simulink model "test_bu01_2018b_tuning"  (R2018b)
settings: Solver=FixedStepAuto  StartTime=0.0  StopTime=10  FixedStep=0.001  RelTol=1e-3
model workspace (MAT data in the model file):
  B1 = 0.0229925610147
  B2 = -0.371283802987
  B3 = -0.920624315565
  B4 = -0.0418343375444
  B5 = -0.493210333206
  B6 = 0
  B7 = -0.0892006103314
  B8 = -0.433620647544
  Ixx = 0.8
  Iyy = 2.075
  Izz = 1.25
  K = 0.92
  K1 = 0.96
  M1 = [1 1 -1 0.151123095698]
  M2 = [1 0 1 0.728919165533]
  M3 = [-1 0 -1 0]
  M4 = [-1 1 1 0.279370204784]
  M5 = [0 -1 0 0.953177368176]
  M6 = [0 -1 0 -1]
  M7 = [0 -1 0 0.164756597211]
  M8 = [0 -1 0 0.72330475505]
  Mass = 11.5
  b = 0
libraries: simulink x4, vrlib x4, shared6dof x1
(part 2 of 3)

== system test_bu01_2018b_tuning/Plant/bu01_model/动力系统模型/Motor4_TM_N/TMU5KV400 /DCMotor1 ==
  In1 : Inport
  Add : Sum  Inputs=+--
  Add1 : Sum  Inputs=+-
  Add2 : Sum
  Add3 : Sum  Inputs=+-
  Bus Selector : BusSelector  OutputSignals=Um,Tq,Izz
  Bus Creator : BusCreator  Inputs=2
  Constant : Constant  Value=Imzz
  Constant1 : Constant  Value=I0
  Divide : Product  Inputs=*/
  Gain : Gain  Gain=1/L
  Gain1 : Gain  Gain=Km
  Gain3 : Gain  Gain=Kemf
  Gain4 : Gain  Gain=Ra
  Gain5 : Gain  Gain=1/(2*pi)
  Gain6 : Gain  Gain=60
  Integrator : Integrator  InitialCondition=0.0001
  Integrator1 : Integrator  InitialCondition=0.0001
  Multiply : Product
  Multiply1 : Product
  Terminator : Terminator
  Terminator1 : Terminator
  Out1 : Outport
  wires:
  In1/1 -> Bus Selector/1
  Bus Selector/1 -> Multiply/1, Add/1  "<Um>"
  Add/1 -> Gain/1
  Gain/1 -> Integrator/1
  Integrator/1 -> Add3/1, Multiply/2, Bus Creator/1, Gain4/1  "Im"
  Gain1/1 -> Multiply1/1, Add1/1  "Te"
  Integrator1/1 -> Multiply1/2, Gain3/1, Gain5/1  "w"
  Add1/1 -> Divide/1
  Divide/1 -> Integrator1/1
  Gain3/1 -> Add/2  "Ea"
  Gain4/1 -> Add/3
  Bus Selector/2 -> [Tq]  "<Tq>"
  Bus Selector/3 -> Add2/1  "<Izz>"
  Constant/1 -> Add2/2
  Add2/1 -> [J]
  [J] -> Divide/2
  Multiply/1 -> Terminator/1  "Pwin"
  Multiply1/1 -> Terminator1/1  "Pwout"
  Gain5/1 -> Gain6/1  "RPS"
  Gain6/1 -> Bus Creator/2  "RPM"
  Bus Creator/1 -> Out1/1
  [Tq] -> Add1/2
  Add3/1 -> Gain1/1  "Iav"
  Constant1/1 -> Add3/2

== system test_bu01_2018b_tuning/Plant/bu01_model/动力系统模型/Motor5_PF_N/PF70mmDuctFanN/涵道风扇模型  ==
  In1 : Inport
  Bus Creator : BusCreator  Inputs=7
  Bus Selector : BusSelector  OutputSignals=Vb,Wb,Ax,Ns,Pro
  If : If  IfExpression=u1 > 1
  Merge : Merge
  Sum : Sum  Inputs=|+-
  Sum1 : Sum  Inputs=|+-
  Terminator : Terminator
  Va : Sqrt  SaturateOnIntegerOverflow=on
  Va^2 : DotProduct  InputSameDT=on  OutDataTypeStr=Inherit: Inherit via internal rule
  Vha : Sqrt  SaturateOnIntegerOverflow=on
  Vva : DotProduct  InputSameDT=on  OutDataTypeStr=Inherit: Inherit via internal rule
  Vva1 : UnaryMinus
  Vva^2 : Math  Operator=square  SaturateOnIntegerOverflow=on
  "[Uba,Vba,Wba]" : UnaryMinus
  求解涵道风扇气动载荷 : Subsystem  TreatAsAtomicUnit=on
  转速太低无载荷输出 : Subsystem  TreatAsAtomicUnit=on
  Out1 : Outport
  wires:
  Bus Selector/1 -> Sum/1  "<Vb>"
  In1/1 -> Bus Selector/1
  Bus Selector/2 -> Sum/2  "<Wb>"
  Sum/1 -> "[Uba,Vba,Wba]"/1
  "[Uba,Vba,Wba]"/1 -> Bus Creator/1, Vva/1, Va^2/2, Va^2/1  "Vba"
  Bus Selector/3 -> Bus Creator/4, Vva/2  "<Ax>"
  Va^2/1 -> Sum1/1, Va/1
  Vva/1 -> Bus Creator/7, Vva^2/1, Vva1/1  "Vva"
  Vva^2/1 -> Sum1/2
  Sum1/1 -> Vha/1
  Vha/1 -> Bus Creator/2  "Vha"
  Vva1/1 -> Bus Creator/3  "Vva1"
  Bus Selector/4 -> Bus Creator/5, If/1  "<Ns>"
  If/1 -> 求解涵道风扇气动载荷/Action
  If/2 -> 转速太低无载荷输出/Action
  Bus Selector/5 -> Bus Creator/6  "<Pro>"
  Bus Creator/1 -> 求解涵道风扇气动载荷/1(In1)
  求解涵道风扇气动载荷/1(Out1) -> Merge/1  "Fb&Mb"
  转速太低无载荷输出/1(Out1) -> Merge/2  "Fb&Mb"
  Va/1 -> Terminator/1  "Va"
  Merge/1 -> Out1/1  "Fb&Mb"

== system test_bu01_2018b_tuning/Plant/bu01_model/动力系统模型/Motor5_PF_N/PFKV2300/DCMotor ==
  In1 : Inport
  Add : Sum  Inputs=+--
  Add1 : Sum  Inputs=+-
  Add2 : Sum
  Add3 : Sum  Inputs=+-
  Bus Selector : BusSelector  OutputSignals=Um,Tq,Izz
  Bus Creator : BusCreator  Inputs=2
  Constant : Constant  Value=Imzz
  Constant1 : Constant  Value=I0
  Divide : Product  Inputs=*/
  Gain : Gain  Gain=1/L
  Gain1 : Gain  Gain=Km
  Gain3 : Gain  Gain=Kemf
  Gain4 : Gain  Gain=Ra
  Gain5 : Gain  Gain=1/(2*pi)
  Gain6 : Gain  Gain=60
  Integrator : Integrator
  Integrator1 : Integrator
  Multiply : Product
  Multiply1 : Product
  Terminator : Terminator
  Terminator1 : Terminator
  Out1 : Outport
  wires:
  In1/1 -> Bus Selector/1
  Bus Selector/1 -> Multiply/1, Add/1  "<Um>"
  Add/1 -> Gain/1
  Gain/1 -> Integrator/1
  Integrator/1 -> Add3/1, Multiply/2, Bus Creator/1, Gain4/1  "Im"
  Gain1/1 -> Multiply1/1, Add1/1  "Te"
  Integrator1/1 -> Multiply1/2, Gain3/1, Gain5/1  "w"
  Add1/1 -> Divide/1
  Divide/1 -> Integrator1/1
  Gain3/1 -> Add/2  "Ea"
  Gain4/1 -> Add/3
  Bus Selector/2 -> [Tq]  "<Tq>"
  Bus Selector/3 -> Add2/1  "<Izz>"
  Constant/1 -> Add2/2
  Add2/1 -> [J]
  [J] -> Divide/2
  Multiply/1 -> Terminator/1  "Pwin"
  Multiply1/1 -> Terminator1/1  "Pwout"
  Gain5/1 -> Gain6/1  "RPS"
  Gain6/1 -> Bus Creator/2  "RPM"
  Bus Creator/1 -> Out1/1
  [Tq] -> Add1/2
  Add3/1 -> Gain1/1  "Iav"
  Constant1/1 -> Add3/2

== system test_bu01_2018b_tuning/Plant/bu01_model/动力系统模型/Motor6_PF_N/PF70mmDuctFanN/涵道风扇模型  ==
  In1 : Inport
  Bus Creator : BusCreator  Inputs=7
  Bus Selector : BusSelector  OutputSignals=Vb,Wb,Ax,Ns,Pro
  If : If  IfExpression=u1 > 1
  Merge : Merge
  Sum : Sum  Inputs=|+-
  Sum1 : Sum  Inputs=|+-
  Terminator : Terminator
  Va : Sqrt  SaturateOnIntegerOverflow=on
  Va^2 : DotProduct  InputSameDT=on  OutDataTypeStr=Inherit: Inherit via internal rule
  Vha : Sqrt  SaturateOnIntegerOverflow=on
  Vva : DotProduct  InputSameDT=on  OutDataTypeStr=Inherit: Inherit via internal rule
  Vva1 : UnaryMinus
  Vva^2 : Math  Operator=square  SaturateOnIntegerOverflow=on
  "[Uba,Vba,Wba]" : UnaryMinus
  求解涵道风扇气动载荷 : Subsystem  TreatAsAtomicUnit=on
  转速太低无载荷输出 : Subsystem  TreatAsAtomicUnit=on
  Out1 : Outport
  wires:
  Bus Selector/1 -> Sum/1  "<Vb>"
  In1/1 -> Bus Selector/1
  Bus Selector/2 -> Sum/2  "<Wb>"
  Sum/1 -> "[Uba,Vba,Wba]"/1
  "[Uba,Vba,Wba]"/1 -> Bus Creator/1, Vva/1, Va^2/2, Va^2/1  "Vba"
  Bus Selector/3 -> Bus Creator/4, Vva/2  "<Ax>"
  Va^2/1 -> Sum1/1, Va/1
  Vva/1 -> Bus Creator/7, Vva^2/1, Vva1/1  "Vva"
  Vva^2/1 -> Sum1/2
  Sum1/1 -> Vha/1
  Vha/1 -> Bus Creator/2  "Vha"
  Vva1/1 -> Bus Creator/3  "Vva1"
  Bus Selector/4 -> Bus Creator/5, If/1  "<Ns>"
  If/1 -> 求解涵道风扇气动载荷/Action
  If/2 -> 转速太低无载荷输出/Action
  Bus Selector/5 -> Bus Creator/6  "<Pro>"
  Bus Creator/1 -> 求解涵道风扇气动载荷/1(In1)
  求解涵道风扇气动载荷/1(Out1) -> Merge/1  "Fb&Mb"
  转速太低无载荷输出/1(Out1) -> Merge/2  "Fb&Mb"
  Va/1 -> Terminator/1  "Va"
  Merge/1 -> Out1/1  "Fb&Mb"

== system test_bu01_2018b_tuning/Plant/bu01_model/动力系统模型/Motor6_PF_N/PFKV2300/DCMotor ==
  In1 : Inport
  Add : Sum  Inputs=+--
  Add1 : Sum  Inputs=+-
  Add2 : Sum
  Add3 : Sum  Inputs=+-
  Bus Selector : BusSelector  OutputSignals=Um,Tq,Izz
  Bus Creator : BusCreator  Inputs=2
  Constant : Constant  Value=Imzz
  Constant1 : Constant  Value=I0
  Divide : Product  Inputs=*/
  Gain : Gain  Gain=1/L
  Gain1 : Gain  Gain=Km
  Gain3 : Gain  Gain=Kemf
  Gain4 : Gain  Gain=Ra
  Gain5 : Gain  Gain=1/(2*pi)
  Gain6 : Gain  Gain=60
  Integrator : Integrator
  Integrator1 : Integrator
  Multiply : Product
  Multiply1 : Product
  Terminator : Terminator
  Terminator1 : Terminator
  Out1 : Outport
  wires:
  In1/1 -> Bus Selector/1
  Bus Selector/1 -> Multiply/1, Add/1  "<Um>"
  Add/1 -> Gain/1
  Gain/1 -> Integrator/1
  Integrator/1 -> Add3/1, Multiply/2, Bus Creator/1, Gain4/1  "Im"
  Gain1/1 -> Multiply1/1, Add1/1  "Te"
  Integrator1/1 -> Multiply1/2, Gain3/1, Gain5/1  "w"
  Add1/1 -> Divide/1
  Divide/1 -> Integrator1/1
  Gain3/1 -> Add/2  "Ea"
  Gain4/1 -> Add/3
  Bus Selector/2 -> [Tq]  "<Tq>"
  Bus Selector/3 -> Add2/1  "<Izz>"
  Constant/1 -> Add2/2
  Add2/1 -> [J]
  [J] -> Divide/2
  Multiply/1 -> Terminator/1  "Pwin"
  Multiply1/1 -> Terminator1/1  "Pwout"
  Gain5/1 -> Gain6/1  "RPS"
  Gain6/1 -> Bus Creator/2  "RPM"
  Bus Creator/1 -> Out1/1
  [Tq] -> Add1/2
  Add3/1 -> Gain1/1  "Iav"
  Constant1/1 -> Add3/2

== system test_bu01_2018b_tuning/Plant/bu01_model/动力系统模型/Motor7_PF_N/PF70mmDuctFanN/涵道风扇模型  ==
  In1 : Inport
  Bus Creator : BusCreator  Inputs=7
  Bus Selector : BusSelector  OutputSignals=Vb,Wb,Ax,Ns,Pro
  If : If  IfExpression=u1 > 1
  Merge : Merge
  Sum : Sum  Inputs=|+-
  Sum1 : Sum  Inputs=|+-
  Terminator : Terminator
  Va : Sqrt  SaturateOnIntegerOverflow=on
  Va^2 : DotProduct  InputSameDT=on  OutDataTypeStr=Inherit: Inherit via internal rule
  Vha : Sqrt  SaturateOnIntegerOverflow=on
  Vva : DotProduct  InputSameDT=on  OutDataTypeStr=Inherit: Inherit via internal rule
  Vva1 : UnaryMinus
  Vva^2 : Math  Operator=square  SaturateOnIntegerOverflow=on
  "[Uba,Vba,Wba]" : UnaryMinus
  求解涵道风扇气动载荷 : Subsystem  TreatAsAtomicUnit=on
  转速太低无载荷输出 : Subsystem  TreatAsAtomicUnit=on
  Out1 : Outport
  wires:
  Bus Selector/1 -> Sum/1  "<Vb>"
  In1/1 -> Bus Selector/1
  Bus Selector/2 -> Sum/2  "<Wb>"
  Sum/1 -> "[Uba,Vba,Wba]"/1
  "[Uba,Vba,Wba]"/1 -> Bus Creator/1, Vva/1, Va^2/2, Va^2/1  "Vba"
  Bus Selector/3 -> Bus Creator/4, Vva/2  "<Ax>"
  Va^2/1 -> Sum1/1, Va/1
  Vva/1 -> Bus Creator/7, Vva^2/1, Vva1/1  "Vva"
  Vva^2/1 -> Sum1/2
  Sum1/1 -> Vha/1
  Vha/1 -> Bus Creator/2  "Vha"
  Vva1/1 -> Bus Creator/3  "Vva1"
  Bus Selector/4 -> Bus Creator/5, If/1  "<Ns>"
  If/1 -> 求解涵道风扇气动载荷/Action
  If/2 -> 转速太低无载荷输出/Action
  Bus Selector/5 -> Bus Creator/6  "<Pro>"
  Bus Creator/1 -> 求解涵道风扇气动载荷/1(In1)
  求解涵道风扇气动载荷/1(Out1) -> Merge/1  "Fb&Mb"
  转速太低无载荷输出/1(Out1) -> Merge/2  "Fb&Mb"
  Va/1 -> Terminator/1  "Va"
  Merge/1 -> Out1/1  "Fb&Mb"

== system test_bu01_2018b_tuning/Plant/bu01_model/动力系统模型/Motor7_PF_N/PFKV2300/DCMotor ==
  In1 : Inport
  Add : Sum  Inputs=+--
  Add1 : Sum  Inputs=+-
  Add2 : Sum
  Add3 : Sum  Inputs=+-
  Bus Selector : BusSelector  OutputSignals=Um,Tq,Izz
  Bus Creator : BusCreator  Inputs=2
  Constant : Constant  Value=Imzz
  Constant1 : Constant  Value=I0
  Divide : Product  Inputs=*/
  Gain : Gain  Gain=1/L
  Gain1 : Gain  Gain=Km
  Gain3 : Gain  Gain=Kemf
  Gain4 : Gain  Gain=Ra
  Gain5 : Gain  Gain=1/(2*pi)
  Gain6 : Gain  Gain=60
  Integrator : Integrator
  Integrator1 : Integrator
  Multiply : Product
  Multiply1 : Product
  Terminator : Terminator
  Terminator1 : Terminator
  Out1 : Outport
  wires:
  In1/1 -> Bus Selector/1
  Bus Selector/1 -> Multiply/1, Add/1  "<Um>"
  Add/1 -> Gain/1
  Gain/1 -> Integrator/1
  Integrator/1 -> Add3/1, Multiply/2, Bus Creator/1, Gain4/1  "Im"
  Gain1/1 -> Multiply1/1, Add1/1  "Te"
  Integrator1/1 -> Multiply1/2, Gain3/1, Gain5/1  "w"
  Add1/1 -> Divide/1
  Divide/1 -> Integrator1/1
  Gain3/1 -> Add/2  "Ea"
  Gain4/1 -> Add/3
  Bus Selector/2 -> [Tq]  "<Tq>"
  Bus Selector/3 -> Add2/1  "<Izz>"
  Constant/1 -> Add2/2
  Add2/1 -> [J]
  [J] -> Divide/2
  Multiply/1 -> Terminator/1  "Pwin"
  Multiply1/1 -> Terminator1/1  "Pwout"
  Gain5/1 -> Gain6/1  "RPS"
  Gain6/1 -> Bus Creator/2  "RPM"
  Bus Creator/1 -> Out1/1
  [Tq] -> Add1/2
  Add3/1 -> Gain1/1  "Iav"
  Constant1/1 -> Add3/2

== system test_bu01_2018b_tuning/Plant/bu01_model/动力系统模型/Motor8_PF_N/PF70mmDuctFanN/涵道风扇模型  ==
  In1 : Inport
  Bus Creator : BusCreator  Inputs=7
  Bus Selector : BusSelector  OutputSignals=Vb,Wb,Ax,Ns,Pro
  If : If  IfExpression=u1 > 1
  Merge : Merge
  Sum : Sum  Inputs=|+-
  Sum1 : Sum  Inputs=|+-
  Terminator : Terminator
  Va : Sqrt  SaturateOnIntegerOverflow=on
  Va^2 : DotProduct  InputSameDT=on  OutDataTypeStr=Inherit: Inherit via internal rule
  Vha : Sqrt  SaturateOnIntegerOverflow=on
  Vva : DotProduct  InputSameDT=on  OutDataTypeStr=Inherit: Inherit via internal rule
  Vva1 : UnaryMinus
  Vva^2 : Math  Operator=square  SaturateOnIntegerOverflow=on
  "[Uba,Vba,Wba]" : UnaryMinus
  求解涵道风扇气动载荷 : Subsystem  TreatAsAtomicUnit=on
  转速太低无载荷输出 : Subsystem  TreatAsAtomicUnit=on
  Out1 : Outport
  wires:
  Merge/1 -> Out1/1  "Fb&Mb"
  Va/1 -> Terminator/1  "Va"
  转速太低无载荷输出/1(Out1) -> Merge/2  "Fb&Mb"
  求解涵道风扇气动载荷/1(Out1) -> Merge/1  "Fb&Mb"
  Bus Creator/1 -> 求解涵道风扇气动载荷/1(In1)
  Bus Selector/5 -> Bus Creator/6  "<Pro>"
  If/2 -> 转速太低无载荷输出/Action
  If/1 -> 求解涵道风扇气动载荷/Action
  Bus Selector/4 -> If/1, Bus Creator/5  "<Ns>"
  Vva1/1 -> Bus Creator/3  "Vva1"
  Vha/1 -> Bus Creator/2  "Vha"
  Sum1/1 -> Vha/1
  Vva^2/1 -> Sum1/2
  Vva/1 -> Vva1/1, Vva^2/1, Bus Creator/7  "Vva"
  Va^2/1 -> Va/1, Sum1/1
  Bus Selector/3 -> Vva/2, Bus Creator/4  "<Ax>"
  "[Uba,Vba,Wba]"/1 -> Va^2/1, Va^2/2, Vva/1, Bus Creator/1  "Vba"
  Sum/1 -> "[Uba,Vba,Wba]"/1
  Bus Selector/2 -> Sum/2  "<Wb>"
  In1/1 -> Bus Selector/1
  Bus Selector/1 -> Sum/1  "<Vb>"

== system test_bu01_2018b_tuning/Plant/bu01_model/动力系统模型/Motor8_PF_N/PFKV2300/DCMotor ==
  In1 : Inport
  Add : Sum  Inputs=+--
  Add1 : Sum  Inputs=+-
  Add2 : Sum
  Add3 : Sum  Inputs=+-
  Bus Selector : BusSelector  OutputSignals=Um,Tq,Izz
  Bus Creator : BusCreator  Inputs=2
  Constant : Constant  Value=Imzz
  Constant1 : Constant  Value=I0
  Divide : Product  Inputs=*/
  Gain : Gain  Gain=1/L
  Gain1 : Gain  Gain=Km
  Gain3 : Gain  Gain=Kemf
  Gain4 : Gain  Gain=Ra
  Gain5 : Gain  Gain=1/(2*pi)
  Gain6 : Gain  Gain=60
  Integrator : Integrator
  Integrator1 : Integrator
  Multiply : Product
  Multiply1 : Product
  Terminator : Terminator
  Terminator1 : Terminator
  Out1 : Outport
  wires:
  Constant1/1 -> Add3/2
  Add3/1 -> Gain1/1  "Iav"
  [Tq] -> Add1/2
  Bus Creator/1 -> Out1/1
  Gain6/1 -> Bus Creator/2  "RPM"
  Gain5/1 -> Gain6/1  "RPS"
  Multiply1/1 -> Terminator1/1  "Pwout"
  Multiply/1 -> Terminator/1  "Pwin"
  [J] -> Divide/2
  Add2/1 -> [J]
  Constant/1 -> Add2/2
  Bus Selector/3 -> Add2/1  "<Izz>"
  Bus Selector/2 -> [Tq]  "<Tq>"
  Gain4/1 -> Add/3
  Gain3/1 -> Add/2  "Ea"
  Divide/1 -> Integrator1/1
  Add1/1 -> Divide/1
  Integrator1/1 -> Gain5/1, Gain3/1, Multiply1/2  "w"
  Gain1/1 -> Add1/1, Multiply1/1  "Te"
  Integrator/1 -> Gain4/1, Bus Creator/1, Multiply/2, Add3/1  "Im"
  Gain/1 -> Integrator/1
  Add/1 -> Gain/1
  Bus Selector/1 -> Add/1, Multiply/1  "<Um>"
  In1/1 -> Bus Selector/1

== system test_bu01_2018b_tuning/Plant/bu01_model/动力系统模型/Motor1_TM_P/TM1654P /螺旋桨模型/不做坐标转换 ==
  F_M : Inport
  Azb : Inport  Port=2
  Action Port : ActionPort  ActionType=then
  Bus Selector1 : BusSelector  OutputSignals=Fxp,Fyp,Fzp,Mxp,Myp,Mzp
  Bus Creator : BusCreator  Inputs=2
  Gain : Gain  Gain=Fratio
  Gain1 : Gain  Gain=Mratio
  Matrix Multiply : Product
  Matrix Multiply1 : Product
  Mux : Mux  Inputs=3
  Mux1 : Mux  Inputs=3
  Out1 : Outport
  wires:
  Bus Selector1/5 -> Mux1/2  "<Myp>"
  Bus Selector1/1 -> Mux/1  "<Fxp>"
  Mux/1 -> Matrix Multiply/2  "F"
  Bus Selector1/4 -> Mux1/1  "<Mxp>"
  Bus Selector1/2 -> Mux/2  "<Fyp>"
  F_M/1 -> Bus Selector1/1
  Mux1/1 -> Matrix Multiply1/2  "M"
  Bus Selector1/6 -> Mux1/3  "<Mzp>"
  Bus Selector1/3 -> Mux/3  "<Fzp>"
  Azb/1 -> Matrix Multiply1/1, Matrix Multiply/1
  Bus Creator/1 -> Out1/1
  Matrix Multiply/1 -> Gain/1
  Gain/1 -> Bus Creator/1  "Fb"
  Matrix Multiply1/1 -> Gain1/1
  Gain1/1 -> Bus Creator/2  "Mb"

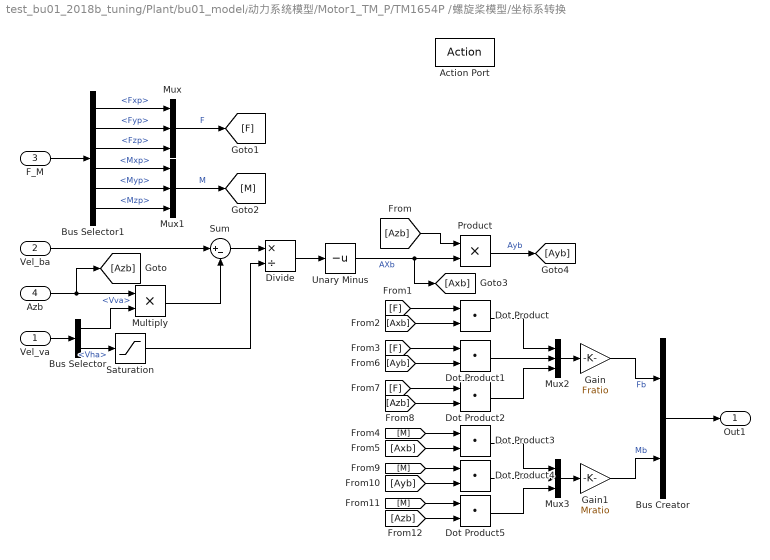
== system test_bu01_2018b_tuning/Plant/bu01_model/动力系统模型/Motor1_TM_P/TM1654P /螺旋桨模型/坐标系转换 ==
  Vel_va : Inport
  Vel_ba : Inport  Port=2
  F_M : Inport  Port=3
  Azb : Inport  Port=4
  Action Port : ActionPort  ActionType=else
  Bus Selector : BusSelector  OutputSignals=Vva,Vha
  Bus Selector1 : BusSelector  OutputSignals=Fxp,Fyp,Fzp,Mxp,Myp,Mzp
  Bus Creator : BusCreator  Inputs=2
  Divide : Product  Inputs=*/
  Dot Product{,1..5} (6 alike) : DotProduct  InputSameDT=on  OutDataTypeStr=Inherit: Inherit via internal rule
  Gain : Gain  Gain=Fratio
  Gain1 : Gain  Gain=Mratio
  Multiply : Product
  Mux{,1..3} (4 alike) : Mux  Inputs=3
  Product : Product
  Saturation : Saturate  UpperLimit=inf  LowerLimit=eps
  Sum : Sum  Inputs=|+-
  Unary Minus : UnaryMinus
  Out1 : Outport
  wires:
  Azb/1 -> [Azb], Multiply/1
  Vel_va/1 -> Bus Selector/1
  Bus Selector/1 -> Multiply/2  "<Vva>"
  Vel_ba/1 -> Sum/1
  Multiply/1 -> Sum/2
  Sum/1 -> Divide/1
  Divide/1 -> Unary Minus/1
  Unary Minus/1 -> [Axb], Product/2  "AXb"
  [Azb] -> Product/1
  Product/1 -> [Ayb]  "Ayb"
  F_M/1 -> Bus Selector1/1
  Bus Selector1/1 -> Mux/1  "<Fxp>"
  Bus Selector1/3 -> Mux/3  "<Fzp>"
  Bus Selector1/2 -> Mux/2  "<Fyp>"
  Mux/1 -> [F]  "F"
  Bus Selector1/4 -> Mux1/1  "<Mxp>"
  Bus Selector1/5 -> Mux1/2  "<Myp>"
  Bus Selector1/6 -> Mux1/3  "<Mzp>"
  Mux1/1 -> [M]  "M"
  Dot Product/1 -> Mux2/1
  [M] -> Dot Product3/1
  [Axb] -> Dot Product3/2
  Dot Product3/1 -> Mux3/1
  [F] -> Dot Product/1
  [Axb] -> Dot Product/2
  [Ayb] -> Dot Product1/2
  Dot Product1/1 -> Mux2/2
  [F] -> Dot Product1/1
  [Azb] -> Dot Product2/2
  Dot Product2/1 -> Mux2/3
  [F] -> Dot Product2/1
  Mux2/1 -> Gain/1
  Dot Product4/1 -> Mux3/2
  [M] -> Dot Product4/1
  [Ayb] -> Dot Product4/2
  Dot Product5/1 -> Mux3/3
  [M] -> Dot Product5/1
  [Azb] -> Dot Product5/2
  Mux3/1 -> Gain1/1
  Gain1/1 -> Bus Creator/2  "Mb"
  Gain/1 -> Bus Creator/1  "Fb"
  Bus Creator/1 -> Out1/1
  Bus Selector/2 -> Saturation/1  "<Vha>"
  Saturation/1 -> Divide/2

== system test_bu01_2018b_tuning/Plant/bu01_model/动力系统模型/Motor1_TM_P/TM1654P /螺旋桨模型/螺旋桨气动 ==
  V : Inport
  Ns : Inport  Port=2
  density : Inport  Port=3
  Abs : Abs
  Bus Selector : BusSelector  OutputSignals=Vva,Vha
  Bus Selector1 : BusSelector  OutputSignals=Mzp
  Bus Creator : BusCreator  Inputs=2
  Bus Creator1 : BusCreator  Inputs=6
  Constant : Constant  Value=D
  Constant1 : Constant  Value=D
  Constant2 : Constant  Value=4
  Constant3 : Constant  Value=[1;1; 1; D; D; D]
  Demux : Demux  Outputs=6
  Divide : Product  Inputs=*/
  Divide1 : Product  Inputs=*/
  Gain : Gain  Gain=Mratio
  Gain1 : Gain  Gain=2*pi
  Multiply : Product
  Multiply1 : Product  Inputs=4
  Multiply2 : Product
  Multiply3 : Product
  Ns1 : InportShadow  Port=2
  Ns2 : InportShadow  Port=2
  Square : Math  Operator=square  SaturateOnIntegerOverflow=on
  Square1 : Math  Operator=pow  OutputSignalType=real  SaturateOnIntegerOverflow=on
  Terminator : Terminator
  Unary Minus : UnaryMinus
  计算螺旋桨气动系数 : Subsystem
  F_M : Outport
  T_q : Outport  Port=2
  wires:
  V/1 -> Bus Selector/1
  Ns/1 -> Multiply/1
  Constant/1 -> Multiply/2
  Multiply/1 -> Divide1/2, Divide/2
  Bus Selector/2 -> Divide/1  "<Vha>"
  Divide/1 -> Bus Creator/2  "Miu"
  Bus Selector/1 -> Unary Minus/1  "<Vva>"
  Unary Minus/1 -> Divide1/1
  Divide1/1 -> Bus Creator/1  "Lumda"
  Bus Creator/1 -> 计算螺旋桨气动系数/1(In1)
  Ns1/1 -> Square/1
  Constant1/1 -> Square1/1
  Constant2/1 -> Square1/2
  Square/1 -> Multiply1/2
  Square1/1 -> Multiply1/3
  Constant3/1 -> Multiply2/1
  Multiply2/1 -> Demux/1
  Demux/1 -> Bus Creator1/1  "Fxp"
  Demux/2 -> Bus Creator1/2  "Fyp"
  Demux/3 -> Bus Creator1/3  "Fzp"
  Demux/4 -> Bus Creator1/4  "Mxp"
  Demux/5 -> Bus Creator1/5  "Myp"
  Demux/6 -> Bus Creator1/6  "Mzp"
  Bus Creator1/1 -> F_M/1, Bus Selector1/1
  Bus Selector1/1 -> Abs/1  "<Mzp>"
  Abs/1 -> Gain/1
  Gain/1 -> T_q/1, Multiply3/1  "Tq"
  Ns2/1 -> Multiply3/2
  Multiply3/1 -> Gain1/1
  Gain1/1 -> Terminator/1  "power"
  density/1 -> Multiply1/4
  计算螺旋桨气动系数/1(Out1) -> Multiply1/1
  Multiply1/1 -> Multiply2/2

== system test_bu01_2018b_tuning/Plant/bu01_model/动力系统模型/Motor2_TM_N/TM1654N /螺旋桨模型/不做坐标转换 ==
  F_M : Inport
  Azb : Inport  Port=2
  Action Port : ActionPort  ActionType=then
  Bus Selector1 : BusSelector  OutputSignals=Fxp,Fyp,Fzp,Mxp,Myp,Mzp
  Bus Creator : BusCreator  Inputs=2
  Gain : Gain  Gain=Fratio
  Gain1 : Gain  Gain=Mratio
  Matrix Multiply : Product
  Matrix Multiply1 : Product
  Mux : Mux  Inputs=3
  Mux1 : Mux  Inputs=3
  Out1 : Outport
  wires:
  Bus Selector1/5 -> Mux1/2  "<Myp>"
  Bus Selector1/1 -> Mux/1  "<Fxp>"
  Mux/1 -> Matrix Multiply/2  "F"
  Bus Selector1/4 -> Mux1/1  "<Mxp>"
  Bus Selector1/2 -> Mux/2  "<Fyp>"
  F_M/1 -> Bus Selector1/1
  Mux1/1 -> Matrix Multiply1/2  "M"
  Bus Selector1/6 -> Mux1/3  "<Mzp>"
  Bus Selector1/3 -> Mux/3  "<Fzp>"
  Azb/1 -> Matrix Multiply1/1, Matrix Multiply/1
  Bus Creator/1 -> Out1/1
  Matrix Multiply/1 -> Gain/1
  Gain/1 -> Bus Creator/1  "Fb"
  Matrix Multiply1/1 -> Gain1/1
  Gain1/1 -> Bus Creator/2  "Mb"

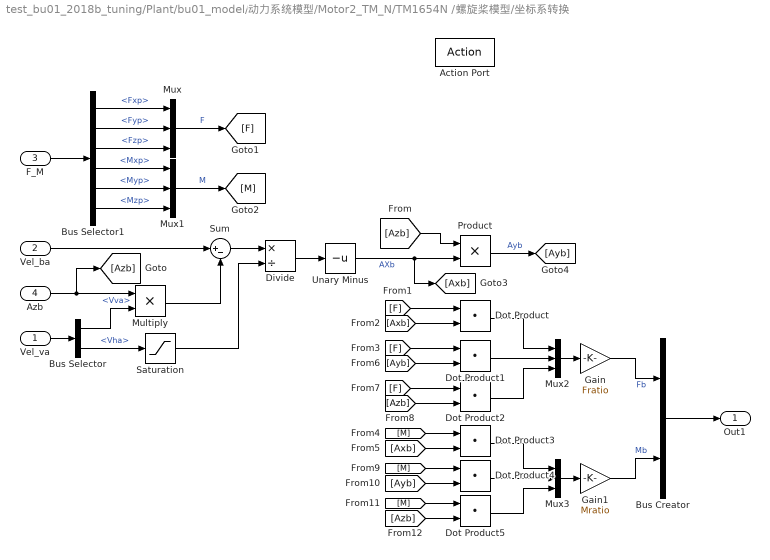
== system test_bu01_2018b_tuning/Plant/bu01_model/动力系统模型/Motor2_TM_N/TM1654N /螺旋桨模型/坐标系转换 ==
  Vel_va : Inport
  Vel_ba : Inport  Port=2
  F_M : Inport  Port=3
  Azb : Inport  Port=4
  Action Port : ActionPort  ActionType=else
  Bus Selector : BusSelector  OutputSignals=Vva,Vha
  Bus Selector1 : BusSelector  OutputSignals=Fxp,Fyp,Fzp,Mxp,Myp,Mzp
  Bus Creator : BusCreator  Inputs=2
  Divide : Product  Inputs=*/
  Dot Product{,1..5} (6 alike) : DotProduct  InputSameDT=on  OutDataTypeStr=Inherit: Inherit via internal rule
  Gain : Gain  Gain=Fratio
  Gain1 : Gain  Gain=Mratio
  Multiply : Product
  Mux{,1..3} (4 alike) : Mux  Inputs=3
  Product : Product
  Saturation : Saturate  UpperLimit=inf  LowerLimit=eps
  Sum : Sum  Inputs=|+-
  Unary Minus : UnaryMinus
  Out1 : Outport
  wires:
  Azb/1 -> [Azb], Multiply/1
  Vel_va/1 -> Bus Selector/1
  Bus Selector/1 -> Multiply/2  "<Vva>"
  Vel_ba/1 -> Sum/1
  Multiply/1 -> Sum/2
  Sum/1 -> Divide/1
  Divide/1 -> Unary Minus/1
  Unary Minus/1 -> [Axb], Product/2  "AXb"
  [Azb] -> Product/1
  Product/1 -> [Ayb]  "Ayb"
  F_M/1 -> Bus Selector1/1
  Bus Selector1/1 -> Mux/1  "<Fxp>"
  Bus Selector1/3 -> Mux/3  "<Fzp>"
  Bus Selector1/2 -> Mux/2  "<Fyp>"
  Mux/1 -> [F]  "F"
  Bus Selector1/4 -> Mux1/1  "<Mxp>"
  Bus Selector1/5 -> Mux1/2  "<Myp>"
  Bus Selector1/6 -> Mux1/3  "<Mzp>"
  Mux1/1 -> [M]  "M"
  Dot Product/1 -> Mux2/1
  [M] -> Dot Product3/1
  [Axb] -> Dot Product3/2
  Dot Product3/1 -> Mux3/1
  [F] -> Dot Product/1
  [Axb] -> Dot Product/2
  [Ayb] -> Dot Product1/2
  Dot Product1/1 -> Mux2/2
  [F] -> Dot Product1/1
  [Azb] -> Dot Product2/2
  Dot Product2/1 -> Mux2/3
  [F] -> Dot Product2/1
  Mux2/1 -> Gain/1
  Dot Product4/1 -> Mux3/2
  [M] -> Dot Product4/1
  [Ayb] -> Dot Product4/2
  Dot Product5/1 -> Mux3/3
  [M] -> Dot Product5/1
  [Azb] -> Dot Product5/2
  Mux3/1 -> Gain1/1
  Gain1/1 -> Bus Creator/2  "Mb"
  Gain/1 -> Bus Creator/1  "Fb"
  Bus Creator/1 -> Out1/1
  Bus Selector/2 -> Saturation/1  "<Vha>"
  Saturation/1 -> Divide/2

== system test_bu01_2018b_tuning/Plant/bu01_model/动力系统模型/Motor2_TM_N/TM1654N /螺旋桨模型/螺旋桨气动 ==
  V : Inport
  Ns : Inport  Port=2
  density : Inport  Port=3
  Abs : Abs
  Bus Selector : BusSelector  OutputSignals=Vva,Vha
  Bus Selector1 : BusSelector  OutputSignals=Mzp
  Bus Creator : BusCreator  Inputs=2
  Bus Creator1 : BusCreator  Inputs=6
  Constant : Constant  Value=D
  Constant1 : Constant  Value=D
  Constant2 : Constant  Value=4
  Constant3 : Constant  Value=[1;-1; 1; -D; D; -D]
  Demux : Demux  Outputs=6
  Divide : Product  Inputs=*/
  Divide1 : Product  Inputs=*/
  Gain : Gain  Gain=Mratio
  Gain1 : Gain  Gain=2*pi
  Multiply : Product
  Multiply1 : Product  Inputs=4
  Multiply2 : Product
  Multiply3 : Product
  Ns1 : InportShadow  Port=2
  Ns2 : InportShadow  Port=2
  Square : Math  Operator=square  SaturateOnIntegerOverflow=on
  Square1 : Math  Operator=pow  OutputSignalType=real  SaturateOnIntegerOverflow=on
  Terminator : Terminator
  Unary Minus : UnaryMinus
  计算螺旋桨气动系数 : Subsystem
  F_M : Outport
  T_q : Outport  Port=2
  wires:
  V/1 -> Bus Selector/1
  Ns/1 -> Multiply/1
  Constant/1 -> Multiply/2
  Multiply/1 -> Divide1/2, Divide/2
  Bus Selector/2 -> Divide/1  "<Vha>"
  Divide/1 -> Bus Creator/2  "Miu"
  Bus Selector/1 -> Unary Minus/1  "<Vva>"
  Unary Minus/1 -> Divide1/1
  Divide1/1 -> Bus Creator/1  "Lumda"
  Bus Creator/1 -> 计算螺旋桨气动系数/1(In1)
  Ns1/1 -> Square/1
  Constant1/1 -> Square1/1
  Constant2/1 -> Square1/2
  Square/1 -> Multiply1/2
  Square1/1 -> Multiply1/3
  Constant3/1 -> Multiply2/1
  Multiply2/1 -> Demux/1
  Demux/1 -> Bus Creator1/1  "Fxp"
  Demux/2 -> Bus Creator1/2  "Fyp"
  Demux/3 -> Bus Creator1/3  "Fzp"
  Demux/4 -> Bus Creator1/4  "Mxp"
  Demux/5 -> Bus Creator1/5  "Myp"
  Demux/6 -> Bus Creator1/6  "Mzp"
  Bus Creator1/1 -> F_M/1, Bus Selector1/1
  Bus Selector1/1 -> Abs/1  "<Mzp>"
  Abs/1 -> Gain/1
  Gain/1 -> T_q/1, Multiply3/1  "Tq"
  Ns2/1 -> Multiply3/2
  Multiply3/1 -> Gain1/1
  Gain1/1 -> Terminator/1  "power"
  density/1 -> Multiply1/4
  计算螺旋桨气动系数/1(Out1) -> Multiply1/1
  Multiply1/1 -> Multiply2/2

== system test_bu01_2018b_tuning/Plant/bu01_model/动力系统模型/Motor3_TM_P/TM1654P /螺旋桨模型/不做坐标转换 ==
  F_M : Inport
  Azb : Inport  Port=2
  Action Port : ActionPort  ActionType=then
  Bus Selector1 : BusSelector  OutputSignals=Fxp,Fyp,Fzp,Mxp,Myp,Mzp
  Bus Creator : BusCreator  Inputs=2
  Gain : Gain  Gain=Fratio
  Gain1 : Gain  Gain=Mratio
  Matrix Multiply : Product
  Matrix Multiply1 : Product
  Mux : Mux  Inputs=3
  Mux1 : Mux  Inputs=3
  Out1 : Outport
  wires:
  Bus Selector1/5 -> Mux1/2  "<Myp>"
  Bus Selector1/1 -> Mux/1  "<Fxp>"
  Mux/1 -> Matrix Multiply/2  "F"
  Bus Selector1/4 -> Mux1/1  "<Mxp>"
  Bus Selector1/2 -> Mux/2  "<Fyp>"
  F_M/1 -> Bus Selector1/1
  Mux1/1 -> Matrix Multiply1/2  "M"
  Bus Selector1/6 -> Mux1/3  "<Mzp>"
  Bus Selector1/3 -> Mux/3  "<Fzp>"
  Azb/1 -> Matrix Multiply1/1, Matrix Multiply/1
  Bus Creator/1 -> Out1/1
  Matrix Multiply/1 -> Gain/1
  Gain/1 -> Bus Creator/1  "Fb"
  Matrix Multiply1/1 -> Gain1/1
  Gain1/1 -> Bus Creator/2  "Mb"

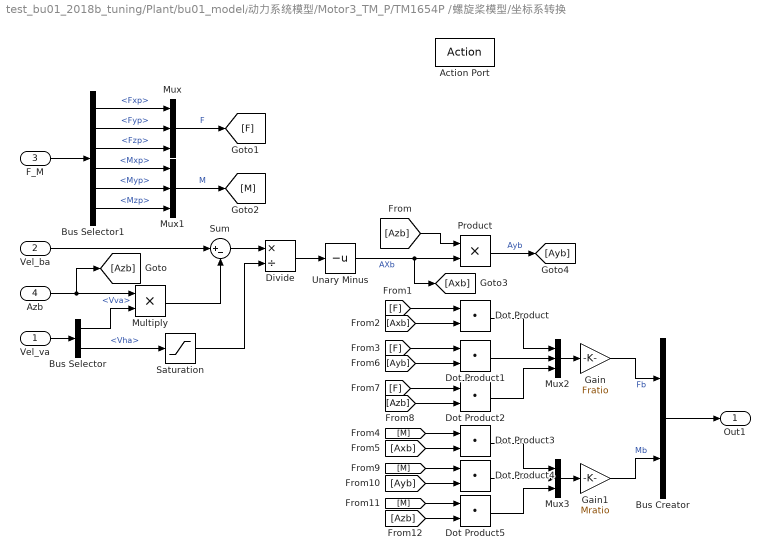
== system test_bu01_2018b_tuning/Plant/bu01_model/动力系统模型/Motor3_TM_P/TM1654P /螺旋桨模型/坐标系转换 ==
  Vel_va : Inport
  Vel_ba : Inport  Port=2
  F_M : Inport  Port=3
  Azb : Inport  Port=4
  Action Port : ActionPort  ActionType=else
  Bus Selector : BusSelector  OutputSignals=Vva,Vha
  Bus Selector1 : BusSelector  OutputSignals=Fxp,Fyp,Fzp,Mxp,Myp,Mzp
  Bus Creator : BusCreator  Inputs=2
  Divide : Product  Inputs=*/
  Dot Product{,1..5} (6 alike) : DotProduct  InputSameDT=on  OutDataTypeStr=Inherit: Inherit via internal rule
  Gain : Gain  Gain=Fratio
  Gain1 : Gain  Gain=Mratio
  Multiply : Product
  Mux{,1..3} (4 alike) : Mux  Inputs=3
  Product : Product
  Saturation : Saturate  UpperLimit=inf  LowerLimit=eps
  Sum : Sum  Inputs=|+-
  Unary Minus : UnaryMinus
  Out1 : Outport
  wires:
  Azb/1 -> [Azb], Multiply/1
  Vel_va/1 -> Bus Selector/1
  Bus Selector/1 -> Multiply/2  "<Vva>"
  Vel_ba/1 -> Sum/1
  Multiply/1 -> Sum/2
  Sum/1 -> Divide/1
  Divide/1 -> Unary Minus/1
  Unary Minus/1 -> [Axb], Product/2  "AXb"
  [Azb] -> Product/1
  Product/1 -> [Ayb]  "Ayb"
  F_M/1 -> Bus Selector1/1
  Bus Selector1/1 -> Mux/1  "<Fxp>"
  Bus Selector1/3 -> Mux/3  "<Fzp>"
  Bus Selector1/2 -> Mux/2  "<Fyp>"
  Mux/1 -> [F]  "F"
  Bus Selector1/4 -> Mux1/1  "<Mxp>"
  Bus Selector1/5 -> Mux1/2  "<Myp>"
  Bus Selector1/6 -> Mux1/3  "<Mzp>"
  Mux1/1 -> [M]  "M"
  Dot Product/1 -> Mux2/1
  [M] -> Dot Product3/1
  [Axb] -> Dot Product3/2
  Dot Product3/1 -> Mux3/1
  [F] -> Dot Product/1
  [Axb] -> Dot Product/2
  [Ayb] -> Dot Product1/2
  Dot Product1/1 -> Mux2/2
  [F] -> Dot Product1/1
  [Azb] -> Dot Product2/2
  Dot Product2/1 -> Mux2/3
  [F] -> Dot Product2/1
  Mux2/1 -> Gain/1
  Dot Product4/1 -> Mux3/2
  [M] -> Dot Product4/1
  [Ayb] -> Dot Product4/2
  Dot Product5/1 -> Mux3/3
  [M] -> Dot Product5/1
  [Azb] -> Dot Product5/2
  Mux3/1 -> Gain1/1
  Gain1/1 -> Bus Creator/2  "Mb"
  Gain/1 -> Bus Creator/1  "Fb"
  Bus Creator/1 -> Out1/1
  Bus Selector/2 -> Saturation/1  "<Vha>"
  Saturation/1 -> Divide/2

== system test_bu01_2018b_tuning/Plant/bu01_model/动力系统模型/Motor3_TM_P/TM1654P /螺旋桨模型/螺旋桨气动 ==
  V : Inport
  Ns : Inport  Port=2
  density : Inport  Port=3
  Abs : Abs
  Bus Selector : BusSelector  OutputSignals=Vva,Vha
  Bus Selector1 : BusSelector  OutputSignals=Mzp
  Bus Creator : BusCreator  Inputs=2
  Bus Creator1 : BusCreator  Inputs=6
  Constant : Constant  Value=D
  Constant1 : Constant  Value=D
  Constant2 : Constant  Value=4
  Constant3 : Constant  Value=[1;1; 1; D; D; D]
  Demux : Demux  Outputs=6
  Divide : Product  Inputs=*/
  Divide1 : Product  Inputs=*/
  Gain : Gain  Gain=Mratio
  Gain1 : Gain  Gain=2*pi
  Multiply : Product
  Multiply1 : Product  Inputs=4
  Multiply2 : Product
  Multiply3 : Product
  Ns1 : InportShadow  Port=2
  Ns2 : InportShadow  Port=2
  Square : Math  Operator=square  SaturateOnIntegerOverflow=on
  Square1 : Math  Operator=pow  OutputSignalType=real  SaturateOnIntegerOverflow=on
  Terminator : Terminator
  Unary Minus : UnaryMinus
  计算螺旋桨气动系数 : Subsystem
  F_M : Outport
  T_q : Outport  Port=2
  wires:
  V/1 -> Bus Selector/1
  Ns/1 -> Multiply/1
  Constant/1 -> Multiply/2
  Multiply/1 -> Divide1/2, Divide/2
  Bus Selector/2 -> Divide/1  "<Vha>"
  Divide/1 -> Bus Creator/2  "Miu"
  Bus Selector/1 -> Unary Minus/1  "<Vva>"
  Unary Minus/1 -> Divide1/1
  Divide1/1 -> Bus Creator/1  "Lumda"
  Bus Creator/1 -> 计算螺旋桨气动系数/1(In1)
  Ns1/1 -> Square/1
  Constant1/1 -> Square1/1
  Constant2/1 -> Square1/2
  Square/1 -> Multiply1/2
  Square1/1 -> Multiply1/3
  Constant3/1 -> Multiply2/1
  Multiply2/1 -> Demux/1
  Demux/1 -> Bus Creator1/1  "Fxp"
  Demux/2 -> Bus Creator1/2  "Fyp"
  Demux/3 -> Bus Creator1/3  "Fzp"
  Demux/4 -> Bus Creator1/4  "Mxp"
  Demux/5 -> Bus Creator1/5  "Myp"
  Demux/6 -> Bus Creator1/6  "Mzp"
  Bus Creator1/1 -> F_M/1, Bus Selector1/1
  Bus Selector1/1 -> Abs/1  "<Mzp>"
  Abs/1 -> Gain/1
  Gain/1 -> T_q/1, Multiply3/1  "Tq"
  Ns2/1 -> Multiply3/2
  Multiply3/1 -> Gain1/1
  Gain1/1 -> Terminator/1  "power"
  density/1 -> Multiply1/4
  计算螺旋桨气动系数/1(Out1) -> Multiply1/1
  Multiply1/1 -> Multiply2/2

== system test_bu01_2018b_tuning/Plant/bu01_model/动力系统模型/Motor4_TM_N/TM1654N /螺旋桨模型/不做坐标转换 ==
  F_M : Inport
  Azb : Inport  Port=2
  Action Port : ActionPort  ActionType=then
  Bus Selector1 : BusSelector  OutputSignals=Fxp,Fyp,Fzp,Mxp,Myp,Mzp
  Bus Creator : BusCreator  Inputs=2
  Gain : Gain  Gain=Fratio
  Gain1 : Gain  Gain=Mratio
  Matrix Multiply : Product
  Matrix Multiply1 : Product
  Mux : Mux  Inputs=3
  Mux1 : Mux  Inputs=3
  Out1 : Outport
  wires:
  Bus Selector1/5 -> Mux1/2  "<Myp>"
  Bus Selector1/1 -> Mux/1  "<Fxp>"
  Mux/1 -> Matrix Multiply/2  "F"
  Bus Selector1/4 -> Mux1/1  "<Mxp>"
  Bus Selector1/2 -> Mux/2  "<Fyp>"
  F_M/1 -> Bus Selector1/1
  Mux1/1 -> Matrix Multiply1/2  "M"
  Bus Selector1/6 -> Mux1/3  "<Mzp>"
  Bus Selector1/3 -> Mux/3  "<Fzp>"
  Azb/1 -> Matrix Multiply1/1, Matrix Multiply/1
  Bus Creator/1 -> Out1/1
  Matrix Multiply/1 -> Gain/1
  Gain/1 -> Bus Creator/1  "Fb"
  Matrix Multiply1/1 -> Gain1/1
  Gain1/1 -> Bus Creator/2  "Mb"

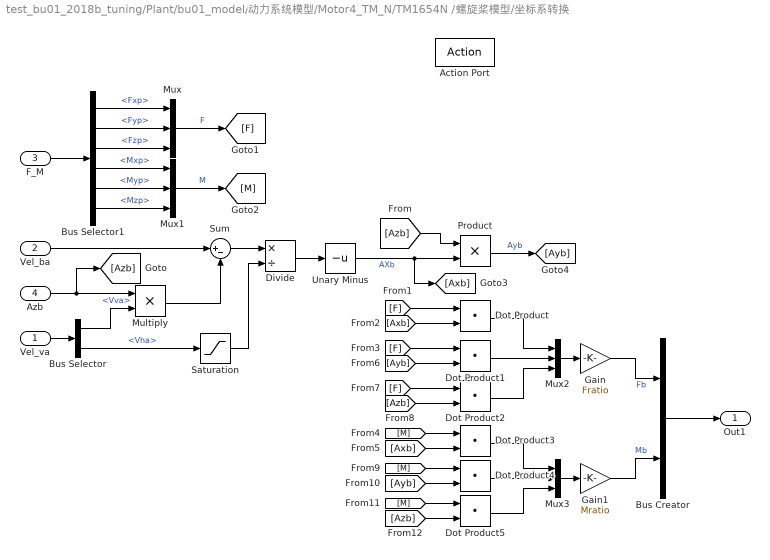
== system test_bu01_2018b_tuning/Plant/bu01_model/动力系统模型/Motor4_TM_N/TM1654N /螺旋桨模型/坐标系转换 ==
  Vel_va : Inport
  Vel_ba : Inport  Port=2
  F_M : Inport  Port=3
  Azb : Inport  Port=4
  Action Port : ActionPort  ActionType=else
  Bus Selector : BusSelector  OutputSignals=Vva,Vha
  Bus Selector1 : BusSelector  OutputSignals=Fxp,Fyp,Fzp,Mxp,Myp,Mzp
  Bus Creator : BusCreator  Inputs=2
  Divide : Product  Inputs=*/
  Dot Product{,1..5} (6 alike) : DotProduct  InputSameDT=on  OutDataTypeStr=Inherit: Inherit via internal rule
  Gain : Gain  Gain=Fratio
  Gain1 : Gain  Gain=Mratio
  Multiply : Product
  Mux{,1..3} (4 alike) : Mux  Inputs=3
  Product : Product
  Saturation : Saturate  UpperLimit=inf  LowerLimit=eps
  Sum : Sum  Inputs=|+-
  Unary Minus : UnaryMinus
  Out1 : Outport
  wires:
  Azb/1 -> [Azb], Multiply/1
  Vel_va/1 -> Bus Selector/1
  Bus Selector/1 -> Multiply/2  "<Vva>"
  Vel_ba/1 -> Sum/1
  Multiply/1 -> Sum/2
  Sum/1 -> Divide/1
  Divide/1 -> Unary Minus/1
  Unary Minus/1 -> [Axb], Product/2  "AXb"
  [Azb] -> Product/1
  Product/1 -> [Ayb]  "Ayb"
  F_M/1 -> Bus Selector1/1
  Bus Selector1/1 -> Mux/1  "<Fxp>"
  Bus Selector1/3 -> Mux/3  "<Fzp>"
  Bus Selector1/2 -> Mux/2  "<Fyp>"
  Mux/1 -> [F]  "F"
  Bus Selector1/4 -> Mux1/1  "<Mxp>"
  Bus Selector1/5 -> Mux1/2  "<Myp>"
  Bus Selector1/6 -> Mux1/3  "<Mzp>"
  Mux1/1 -> [M]  "M"
  Dot Product/1 -> Mux2/1
  [M] -> Dot Product3/1
  [Axb] -> Dot Product3/2
  Dot Product3/1 -> Mux3/1
  [F] -> Dot Product/1
  [Axb] -> Dot Product/2
  [Ayb] -> Dot Product1/2
  Dot Product1/1 -> Mux2/2
  [F] -> Dot Product1/1
  [Azb] -> Dot Product2/2
  Dot Product2/1 -> Mux2/3
  [F] -> Dot Product2/1
  Mux2/1 -> Gain/1
  Dot Product4/1 -> Mux3/2
  [M] -> Dot Product4/1
  [Ayb] -> Dot Product4/2
  Dot Product5/1 -> Mux3/3
  [M] -> Dot Product5/1
  [Azb] -> Dot Product5/2
  Mux3/1 -> Gain1/1
  Gain1/1 -> Bus Creator/2  "Mb"
  Gain/1 -> Bus Creator/1  "Fb"
  Bus Creator/1 -> Out1/1
  Bus Selector/2 -> Saturation/1  "<Vha>"
  Saturation/1 -> Divide/2

== system test_bu01_2018b_tuning/Plant/bu01_model/动力系统模型/Motor4_TM_N/TM1654N /螺旋桨模型/螺旋桨气动 ==
  V : Inport
  Ns : Inport  Port=2
  density : Inport  Port=3
  Abs : Abs
  Bus Selector : BusSelector  OutputSignals=Vva,Vha
  Bus Selector1 : BusSelector  OutputSignals=Mzp
  Bus Creator : BusCreator  Inputs=2
  Bus Creator1 : BusCreator  Inputs=6
  Constant : Constant  Value=D
  Constant1 : Constant  Value=D
  Constant2 : Constant  Value=4
  Constant3 : Constant  Value=[1;-1; 1; -D; D; -D]
  Demux : Demux  Outputs=6
  Divide : Product  Inputs=*/
  Divide1 : Product  Inputs=*/
  Gain : Gain  Gain=Mratio
  Gain1 : Gain  Gain=2*pi
  Multiply : Product
  Multiply1 : Product  Inputs=4
  Multiply2 : Product
  Multiply3 : Product
  Ns1 : InportShadow  Port=2
  Ns2 : InportShadow  Port=2
  Square : Math  Operator=square  SaturateOnIntegerOverflow=on
  Square1 : Math  Operator=pow  OutputSignalType=real  SaturateOnIntegerOverflow=on
  Terminator : Terminator
  Unary Minus : UnaryMinus
  计算螺旋桨气动系数 : Subsystem
  F_M : Outport
  T_q : Outport  Port=2
  wires:
  V/1 -> Bus Selector/1
  Ns/1 -> Multiply/1
  Constant/1 -> Multiply/2
  Multiply/1 -> Divide1/2, Divide/2
  Bus Selector/2 -> Divide/1  "<Vha>"
  Divide/1 -> Bus Creator/2  "Miu"
  Bus Selector/1 -> Unary Minus/1  "<Vva>"
  Unary Minus/1 -> Divide1/1
  Divide1/1 -> Bus Creator/1  "Lumda"
  Bus Creator/1 -> 计算螺旋桨气动系数/1(In1)
  Ns1/1 -> Square/1
  Constant1/1 -> Square1/1
  Constant2/1 -> Square1/2
  Square/1 -> Multiply1/2
  Square1/1 -> Multiply1/3
  Constant3/1 -> Multiply2/1
  Multiply2/1 -> Demux/1
  Demux/1 -> Bus Creator1/1  "Fxp"
  Demux/2 -> Bus Creator1/2  "Fyp"
  Demux/3 -> Bus Creator1/3  "Fzp"
  Demux/4 -> Bus Creator1/4  "Mxp"
  Demux/5 -> Bus Creator1/5  "Myp"
  Demux/6 -> Bus Creator1/6  "Mzp"
  Bus Creator1/1 -> F_M/1, Bus Selector1/1
  Bus Selector1/1 -> Abs/1  "<Mzp>"
  Abs/1 -> Gain/1
  Gain/1 -> T_q/1, Multiply3/1  "Tq"
  Ns2/1 -> Multiply3/2
  Multiply3/1 -> Gain1/1
  Gain1/1 -> Terminator/1  "power"
  density/1 -> Multiply1/4
  计算螺旋桨气动系数/1(Out1) -> Multiply1/1
  Multiply1/1 -> Multiply2/2

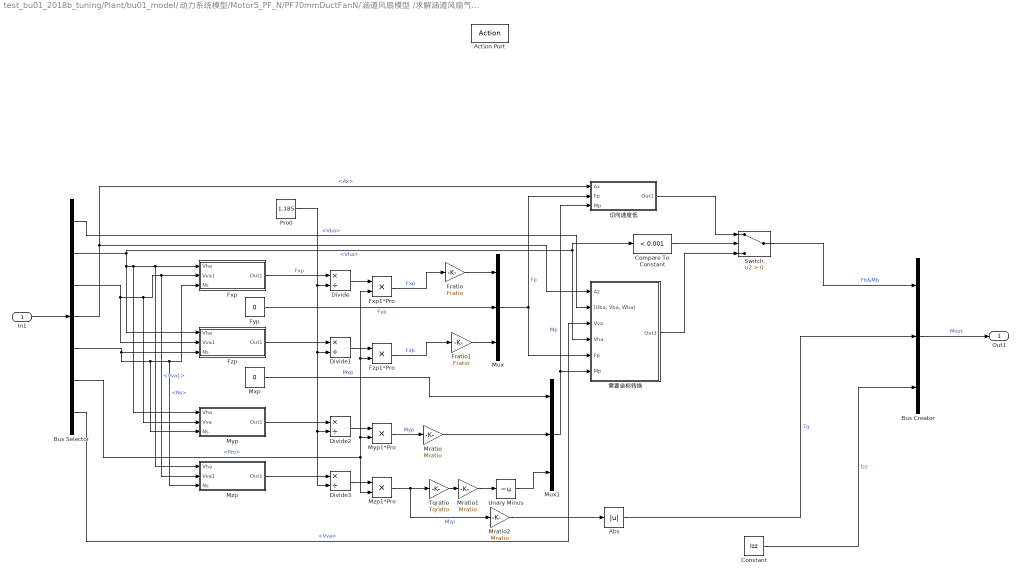
== system test_bu01_2018b_tuning/Plant/bu01_model/动力系统模型/Motor5_PF_N/PF70mmDuctFanN/涵道风扇模型 /求解涵道风扇气动载荷 ==
  In1 : Inport
  Action Port : ActionPort  ActionType=then
  Abs : Abs
  Bus Creator : BusCreator  Inputs=3
  Bus Selector : BusSelector  OutputSignals=Vba,Vha,Vva1,Ax,Ns,Pro,Vva
  Compare To Constant : simulink/Logic and Bit Operations/Compare To Constant  relop=<  const=0.001  OutDataTypeStr=boolean
  Constant : Constant  Value=Izz
  Divide{,1..3} (4 alike) : Product  Inputs=*/
  Fratio : Gain  Gain=Fratio
  Fratio1 : Gain  Gain=Fratio
  Fxp : Subsystem
  Fxp1*Pro : Product
  Fyp : Constant  Value=0
  Fzp : Subsystem
  Fzp1*Pro : Product
  Mratio : Gain  Gain=Mratio
  Mratio1 : Gain  Gain=Mratio
  Mratio2 : Gain  Gain=Mratio
  Mux : Mux  Inputs=3
  Mux1 : Mux  Inputs=3
  Mxp : Constant  Value=0
  Myp : Subsystem
  Myp1*Pro : Product
  Mzp : Subsystem
  Mzp1*Pro : Product
  Pro0 : Constant  Value=1.185
  Switch : Switch  Criteria=u2 > Threshold
  Tqratio : Gain  Gain=Tqratio
  Unary Minus : UnaryMinus
  切向速度低 : Subsystem
  需要坐标转换 : Subsystem
  Out1 : Outport
  wires:
  In1/1 -> Bus Selector/1
  Bus Selector/2 -> Fzp/1(Vha), Myp/1(Vha), Mzp/1(Vha), Fxp/1(Vha), 需要坐标转换/4(Vha), Compare To Constant/1  "<Vha>"
  Bus Selector/3 -> Myp/2(Vva), Mzp/2(Vva1), Fxp/2(Vva1), Fzp/2(Vva1)  "<Vva1>"
  Bus Selector/5 -> Fzp/3(Ns), Myp/3(Ns), Mzp/3(Ns), Fxp/3(Ns)  "<Ns>"
  Fyp/1 -> Mux/2  "Fyp"
  Fxp/1(Out1) -> Divide/1  "Fxp"
  Fzp/1(Out1) -> Divide1/1
  Myp/1(Out1) -> Divide2/1
  Mzp/1(Out1) -> Divide3/1
  Pro0/1 -> Divide3/2, Divide2/2, Divide1/2, Divide/2
  Divide/1 -> Fxp1*Pro/1
  Fxp1*Pro/1 -> Fratio/1  "Fxp"
  Divide1/1 -> Fzp1*Pro/1
  Fzp1*Pro/1 -> Fratio1/1  "Fzp"
  Bus Selector/6 -> Mzp1*Pro/2, Myp1*Pro/2, Fzp1*Pro/2, Fxp1*Pro/2  "<Pro>"
  Divide2/1 -> Myp1*Pro/1
  Myp1*Pro/1 -> Mratio/1  "Myp"
  Divide3/1 -> Mzp1*Pro/1
  Bus Selector/4 -> 需要坐标转换/1(Az), 切向速度低/1(Ax)  "<Ax>"
  Mux/1 -> 需要坐标转换/5(Fp), 切向速度低/2(Fp)  "Fp"
  Mux1/1 -> 需要坐标转换/6(Mp), 切向速度低/3(Mp)  "Mp"
  Bus Selector/1 -> 需要坐标转换/2("[Uba, Vba, Wba]")  "<Vba>"
  Bus Selector/7 -> 需要坐标转换/3(Vva)  "<Vva>"
  Compare To Constant/1 -> Switch/2
  需要坐标转换/1(Out1) -> Switch/3
  Abs/1 -> Bus Creator/2  "Tq"
  Mzp1*Pro/1 -> Mratio2/1, Tqratio/1  "Mzp"
  Fratio/1 -> Mux/1
  Fratio1/1 -> Mux/3
  Tqratio/1 -> Mratio1/1
  Mratio/1 -> Mux1/2
  Mratio2/1 -> Abs/1
  Constant/1 -> Bus Creator/3  "Izz"
  Switch/1 -> Bus Creator/1  "Fb&Mb"
  Bus Creator/1 -> Out1/1  "Mout"
  切向速度低/1(Out1) -> Switch/1
  Mxp/1 -> Mux1/1  "Mxp"
  Mratio1/1 -> Unary Minus/1
  Unary Minus/1 -> Mux1/3

== system test_bu01_2018b_tuning/Plant/bu01_model/动力系统模型/Motor5_PF_N/PF70mmDuctFanN/涵道风扇模型 /转速太低无载荷输出 ==
  Action Port : ActionPort  ActionType=else
  Bus Creator : BusCreator  Inputs=3
  Bus Creator1 : BusCreator  Inputs=2
  Constant : Constant  Value=[0 0 0]
  Constant3 : Constant  Value=[0 0 0]
  Constant6 : Constant  Value=0
  Constant7 : Constant  Value=Izz
  Out1 : Outport
  wires:
  Constant6/1 -> Bus Creator/2  "Tq"
  Constant7/1 -> Bus Creator/3  "Izz"
  Bus Creator/1 -> Out1/1  "Mout"
  Constant/1 -> Bus Creator1/1  "Fb"
  Constant3/1 -> Bus Creator1/2  "Mb"
  Bus Creator1/1 -> Bus Creator/1  "Fb&Mb"

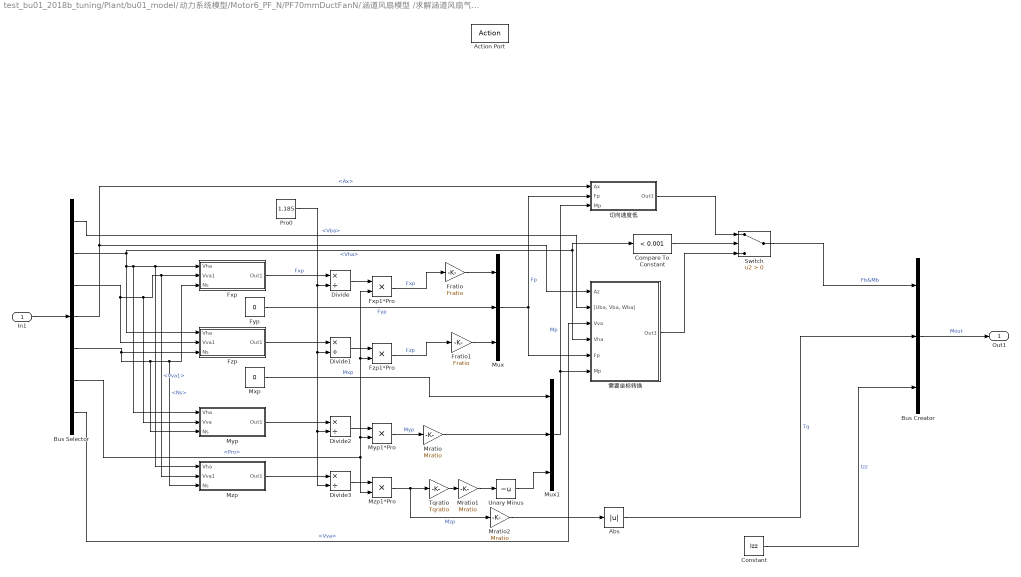
== system test_bu01_2018b_tuning/Plant/bu01_model/动力系统模型/Motor6_PF_N/PF70mmDuctFanN/涵道风扇模型 /求解涵道风扇气动载荷 ==
  In1 : Inport
  Action Port : ActionPort  ActionType=then
  Abs : Abs
  Bus Creator : BusCreator  Inputs=3
  Bus Selector : BusSelector  OutputSignals=Vba,Vha,Vva1,Ax,Ns,Pro,Vva
  Compare To Constant : simulink/Logic and Bit Operations/Compare To Constant  relop=<  const=0.001  OutDataTypeStr=boolean
  Constant : Constant  Value=Izz
  Divide{,1..3} (4 alike) : Product  Inputs=*/
  Fratio : Gain  Gain=Fratio
  Fratio1 : Gain  Gain=Fratio
  Fxp : Subsystem
  Fxp1*Pro : Product
  Fyp : Constant  Value=0
  Fzp : Subsystem
  Fzp1*Pro : Product
  Mratio : Gain  Gain=Mratio
  Mratio1 : Gain  Gain=Mratio
  Mratio2 : Gain  Gain=Mratio
  Mux : Mux  Inputs=3
  Mux1 : Mux  Inputs=3
  Mxp : Constant  Value=0
  Myp : Subsystem
  Myp1*Pro : Product
  Mzp : Subsystem
  Mzp1*Pro : Product
  Pro0 : Constant  Value=1.185
  Switch : Switch  Criteria=u2 > Threshold
  Tqratio : Gain  Gain=Tqratio
  Unary Minus : UnaryMinus
  切向速度低 : Subsystem
  需要坐标转换 : Subsystem
  Out1 : Outport
  wires:
  In1/1 -> Bus Selector/1
  Bus Selector/2 -> Fzp/1(Vha), Myp/1(Vha), Mzp/1(Vha), Fxp/1(Vha), 需要坐标转换/4(Vha), Compare To Constant/1  "<Vha>"
  Bus Selector/3 -> Myp/2(Vva), Mzp/2(Vva1), Fxp/2(Vva1), Fzp/2(Vva1)  "<Vva1>"
  Bus Selector/5 -> Fzp/3(Ns), Myp/3(Ns), Mzp/3(Ns), Fxp/3(Ns)  "<Ns>"
  Fyp/1 -> Mux/2  "Fyp"
  Fxp/1(Out1) -> Divide/1  "Fxp"
  Fzp/1(Out1) -> Divide1/1
  Myp/1(Out1) -> Divide2/1
  Mzp/1(Out1) -> Divide3/1
  Pro0/1 -> Divide3/2, Divide2/2, Divide1/2, Divide/2
  Divide/1 -> Fxp1*Pro/1
  Fxp1*Pro/1 -> Fratio/1  "Fxp"
  Divide1/1 -> Fzp1*Pro/1
  Fzp1*Pro/1 -> Fratio1/1  "Fzp"
  Bus Selector/6 -> Mzp1*Pro/2, Myp1*Pro/2, Fzp1*Pro/2, Fxp1*Pro/2  "<Pro>"
  Divide2/1 -> Myp1*Pro/1
  Myp1*Pro/1 -> Mratio/1  "Myp"
  Divide3/1 -> Mzp1*Pro/1
  Bus Selector/4 -> 需要坐标转换/1(Az), 切向速度低/1(Ax)  "<Ax>"
  Mux/1 -> 需要坐标转换/5(Fp), 切向速度低/2(Fp)  "Fp"
  Mux1/1 -> 需要坐标转换/6(Mp), 切向速度低/3(Mp)  "Mp"
  Bus Selector/1 -> 需要坐标转换/2("[Uba, Vba, Wba]")  "<Vba>"
  Bus Selector/7 -> 需要坐标转换/3(Vva)  "<Vva>"
  Compare To Constant/1 -> Switch/2
  需要坐标转换/1(Out1) -> Switch/3
  Abs/1 -> Bus Creator/2  "Tq"
  Mzp1*Pro/1 -> Mratio2/1, Tqratio/1  "Mzp"
  Fratio/1 -> Mux/1
  Fratio1/1 -> Mux/3
  Tqratio/1 -> Mratio1/1
  Mratio/1 -> Mux1/2
  Mratio2/1 -> Abs/1
  Constant/1 -> Bus Creator/3  "Izz"
  Switch/1 -> Bus Creator/1  "Fb&Mb"
  Bus Creator/1 -> Out1/1  "Mout"
  切向速度低/1(Out1) -> Switch/1
  Mxp/1 -> Mux1/1  "Mxp"
  Mratio1/1 -> Unary Minus/1
  Unary Minus/1 -> Mux1/3

== system test_bu01_2018b_tuning/Plant/bu01_model/动力系统模型/Motor6_PF_N/PF70mmDuctFanN/涵道风扇模型 /转速太低无载荷输出 ==
  Action Port : ActionPort  ActionType=else
  Bus Creator : BusCreator  Inputs=3
  Bus Creator1 : BusCreator  Inputs=2
  Constant : Constant  Value=[0 0 0]
  Constant3 : Constant  Value=[0 0 0]
  Constant6 : Constant  Value=0
  Constant7 : Constant  Value=Izz
  Out1 : Outport
  wires:
  Constant6/1 -> Bus Creator/2  "Tq"
  Constant7/1 -> Bus Creator/3  "Izz"
  Bus Creator/1 -> Out1/1  "Mout"
  Constant/1 -> Bus Creator1/1  "Fb"
  Constant3/1 -> Bus Creator1/2  "Mb"
  Bus Creator1/1 -> Bus Creator/1  "Fb&Mb"

== system test_bu01_2018b_tuning/Plant/bu01_model/动力系统模型/Motor7_PF_N/PF70mmDuctFanN/涵道风扇模型 /求解涵道风扇气动载荷 ==
  In1 : Inport
  Action Port : ActionPort  ActionType=then
  Abs : Abs
  Bus Creator : BusCreator  Inputs=3
  Bus Selector : BusSelector  OutputSignals=Vba,Vha,Vva1,Ax,Ns,Pro,Vva
  Compare To Constant : simulink/Logic and Bit Operations/Compare To Constant  relop=<  const=0.001  OutDataTypeStr=boolean
  Constant : Constant  Value=Izz
  Divide{,1..3} (4 alike) : Product  Inputs=*/
  Fratio : Gain  Gain=Fratio
  Fratio1 : Gain  Gain=Fratio
  Fxp : Subsystem
  Fxp1*Pro : Product
  Fyp : Constant  Value=0
  Fzp : Subsystem
  Fzp1*Pro : Product
  Mratio : Gain  Gain=Mratio
  Mratio1 : Gain  Gain=Mratio
  Mratio2 : Gain  Gain=Mratio
  Mux : Mux  Inputs=3
  Mux1 : Mux  Inputs=3
  Mxp : Constant  Value=0
  Myp : Subsystem
  Myp1*Pro : Product
  Mzp : Subsystem
  Mzp1*Pro : Product
  Pro0 : Constant  Value=1.185
  Switch : Switch  Criteria=u2 > Threshold
  Tqratio : Gain  Gain=Tqratio
  Unary Minus : UnaryMinus
  切向速度低 : Subsystem
  需要坐标转换 : Subsystem
  Out1 : Outport
  wires:
  In1/1 -> Bus Selector/1
  Bus Selector/2 -> Fzp/1(Vha), Myp/1(Vha), Mzp/1(Vha), Fxp/1(Vha), 需要坐标转换/4(Vha), Compare To Constant/1  "<Vha>"
  Bus Selector/3 -> Myp/2(Vva), Mzp/2(Vva1), Fxp/2(Vva1), Fzp/2(Vva1)  "<Vva1>"
  Bus Selector/5 -> Fzp/3(Ns), Myp/3(Ns), Mzp/3(Ns), Fxp/3(Ns)  "<Ns>"
  Fyp/1 -> Mux/2  "Fyp"
  Fxp/1(Out1) -> Divide/1  "Fxp"
  Fzp/1(Out1) -> Divide1/1
  Myp/1(Out1) -> Divide2/1
  Mzp/1(Out1) -> Divide3/1
  Pro0/1 -> Divide3/2, Divide2/2, Divide1/2, Divide/2
  Divide/1 -> Fxp1*Pro/1
  Fxp1*Pro/1 -> Fratio/1  "Fxp"
  Divide1/1 -> Fzp1*Pro/1
  Fzp1*Pro/1 -> Fratio1/1  "Fzp"
  Bus Selector/6 -> Mzp1*Pro/2, Myp1*Pro/2, Fzp1*Pro/2, Fxp1*Pro/2  "<Pro>"
  Divide2/1 -> Myp1*Pro/1
  Myp1*Pro/1 -> Mratio/1  "Myp"
  Divide3/1 -> Mzp1*Pro/1
  Bus Selector/4 -> 需要坐标转换/1(Az), 切向速度低/1(Ax)  "<Ax>"
  Mux/1 -> 需要坐标转换/5(Fp), 切向速度低/2(Fp)  "Fp"
  Mux1/1 -> 需要坐标转换/6(Mp), 切向速度低/3(Mp)  "Mp"
  Bus Selector/1 -> 需要坐标转换/2("[Uba, Vba, Wba]")  "<Vba>"
  Bus Selector/7 -> 需要坐标转换/3(Vva)  "<Vva>"
  Compare To Constant/1 -> Switch/2
  需要坐标转换/1(Out1) -> Switch/3
  Abs/1 -> Bus Creator/2  "Tq"
  Mzp1*Pro/1 -> Mratio2/1, Tqratio/1  "Mzp"
  Fratio/1 -> Mux/1
  Fratio1/1 -> Mux/3
  Tqratio/1 -> Mratio1/1
  Mratio/1 -> Mux1/2
  Mratio2/1 -> Abs/1
  Constant/1 -> Bus Creator/3  "Izz"
  Switch/1 -> Bus Creator/1  "Fb&Mb"
  Bus Creator/1 -> Out1/1  "Mout"
  切向速度低/1(Out1) -> Switch/1
  Mxp/1 -> Mux1/1  "Mxp"
  Mratio1/1 -> Unary Minus/1
  Unary Minus/1 -> Mux1/3

== system test_bu01_2018b_tuning/Plant/bu01_model/动力系统模型/Motor7_PF_N/PF70mmDuctFanN/涵道风扇模型 /转速太低无载荷输出 ==
  Action Port : ActionPort  ActionType=else
  Bus Creator : BusCreator  Inputs=3
  Bus Creator1 : BusCreator  Inputs=2
  Constant : Constant  Value=[0 0 0]
  Constant3 : Constant  Value=[0 0 0]
  Constant6 : Constant  Value=0
  Constant7 : Constant  Value=Izz
  Out1 : Outport
  wires:
  Constant6/1 -> Bus Creator/2  "Tq"
  Constant7/1 -> Bus Creator/3  "Izz"
  Bus Creator/1 -> Out1/1  "Mout"
  Constant/1 -> Bus Creator1/1  "Fb"
  Constant3/1 -> Bus Creator1/2  "Mb"
  Bus Creator1/1 -> Bus Creator/1  "Fb&Mb"

== system test_bu01_2018b_tuning/Plant/bu01_model/动力系统模型/Motor8_PF_N/PF70mmDuctFanN/涵道风扇模型 /求解涵道风扇气动载荷 ==
  In1 : Inport
  Action Port : ActionPort  ActionType=then
  Abs : Abs
  Bus Creator : BusCreator  Inputs=3
  Bus Selector : BusSelector  OutputSignals=Vba,Vha,Vva1,Ax,Ns,Pro,Vva
  Compare To Constant : simulink/Logic and Bit Operations/Compare To Constant  relop=<  const=0.001  OutDataTypeStr=boolean
  Constant : Constant  Value=Izz
  Divide{,1..3} (4 alike) : Product  Inputs=*/
  Fratio : Gain  Gain=Fratio
  Fratio1 : Gain  Gain=Fratio
  Fxp : Subsystem
  Fxp1*Pro : Product
  Fyp : Constant  Value=0
  Fzp : Subsystem
  Fzp1*Pro : Product
  Mratio : Gain  Gain=Mratio
  Mratio1 : Gain  Gain=Mratio
  Mratio2 : Gain  Gain=Mratio
  Mux : Mux  Inputs=3
  Mux1 : Mux  Inputs=3
  Mxp : Constant  Value=0
  Myp : Subsystem
  Myp1*Pro : Product
  Mzp : Subsystem
  Mzp1*Pro : Product
  Pro0 : Constant  Value=1.185
  Switch : Switch  Criteria=u2 > Threshold
  Tqratio : Gain  Gain=Tqratio
  Unary Minus : UnaryMinus
  切向速度低 : Subsystem
  需要坐标转换 : Subsystem
  Out1 : Outport
  wires:
  Unary Minus/1 -> Mux1/3
  Mratio1/1 -> Unary Minus/1
  Mxp/1 -> Mux1/1  "Mxp"
  切向速度低/1(Out1) -> Switch/1
  Bus Creator/1 -> Out1/1  "Mout"
  Switch/1 -> Bus Creator/1  "Fb&Mb"
  Constant/1 -> Bus Creator/3  "Izz"
  Mratio2/1 -> Abs/1
  Mratio/1 -> Mux1/2
  Tqratio/1 -> Mratio1/1
  Fratio1/1 -> Mux/3
  Fratio/1 -> Mux/1
  Mzp1*Pro/1 -> Tqratio/1, Mratio2/1  "Mzp"
  Abs/1 -> Bus Creator/2  "Tq"
  需要坐标转换/1(Out1) -> Switch/3
  Compare To Constant/1 -> Switch/2
  Bus Selector/7 -> 需要坐标转换/3(Vva)  "<Vva>"
  Bus Selector/1 -> 需要坐标转换/2("[Uba, Vba, Wba]")  "<Vba>"
  Mux1/1 -> 切向速度低/3(Mp), 需要坐标转换/6(Mp)  "Mp"
  Mux/1 -> 切向速度低/2(Fp), 需要坐标转换/5(Fp)  "Fp"
  Bus Selector/4 -> 切向速度低/1(Ax), 需要坐标转换/1(Az)  "<Ax>"
  Divide3/1 -> Mzp1*Pro/1
  Myp1*Pro/1 -> Mratio/1  "Myp"
  Divide2/1 -> Myp1*Pro/1
  Bus Selector/6 -> Fxp1*Pro/2, Fzp1*Pro/2, Myp1*Pro/2, Mzp1*Pro/2  "<Pro>"
  Fzp1*Pro/1 -> Fratio1/1  "Fzp"
  Divide1/1 -> Fzp1*Pro/1
  Fxp1*Pro/1 -> Fratio/1  "Fxp"
  Divide/1 -> Fxp1*Pro/1
  Pro0/1 -> Divide/2, Divide1/2, Divide2/2, Divide3/2
  Mzp/1(Out1) -> Divide3/1
  Myp/1(Out1) -> Divide2/1
  Fzp/1(Out1) -> Divide1/1
  Fxp/1(Out1) -> Divide/1  "Fxp"
  Fyp/1 -> Mux/2  "Fyp"
  Bus Selector/5 -> Fxp/3(Ns), Mzp/3(Ns), Myp/3(Ns), Fzp/3(Ns)  "<Ns>"
  Bus Selector/3 -> Fzp/2(Vva1), Fxp/2(Vva1), Mzp/2(Vva1), Myp/2(Vva)  "<Vva1>"
  Bus Selector/2 -> Compare To Constant/1, 需要坐标转换/4(Vha), Fxp/1(Vha), Mzp/1(Vha), Myp/1(Vha), Fzp/1(Vha)  "<Vha>"
  In1/1 -> Bus Selector/1

== system test_bu01_2018b_tuning/Plant/bu01_model/动力系统模型/Motor8_PF_N/PF70mmDuctFanN/涵道风扇模型 /转速太低无载荷输出 ==
  Action Port : ActionPort  ActionType=else
  Bus Creator : BusCreator  Inputs=3
  Bus Creator1 : BusCreator  Inputs=2
  Constant : Constant  Value=[0 0 0]
  Constant3 : Constant  Value=[0 0 0]
  Constant6 : Constant  Value=0
  Constant7 : Constant  Value=Izz
  Out1 : Outport
  wires:
  Bus Creator1/1 -> Bus Creator/1  "Fb&Mb"
  Constant3/1 -> Bus Creator1/2  "Mb"
  Constant/1 -> Bus Creator1/1  "Fb"
  Bus Creator/1 -> Out1/1  "Mout"
  Constant7/1 -> Bus Creator/3  "Izz"
  Constant6/1 -> Bus Creator/2  "Tq"

== system test_bu01_2018b_tuning/Plant/bu01_model/动力系统模型/Motor1_TM_P/TM1654P /螺旋桨模型/螺旋桨气动/计算螺旋桨气动系数 ==
  In1 : Inport
  Bus Selector : BusSelector  OutputSignals=Miu,Lumda
  Mux : Mux  Inputs=6
  计算Cmx : Subsystem
  计算Cmy : Subsystem
  计算Cmz : Subsystem
  计算Ctx : Subsystem  TreatAsAtomicUnit=on
  计算Cty : Subsystem
  计算Ctz : Subsystem
  Out1 : Outport
  wires:
  In1/1 -> Bus Selector/1
  Bus Selector/1 -> 计算Ctz/1(Miu), 计算Cmz/1(Miu), 计算Cmy/1(Miu), 计算Cmx/1(Miu), 计算Cty/1(Miu), 计算Ctx/1(Miu)  "<Miu>"
  Bus Selector/2 -> 计算Cty/2(Lumda), 计算Ctx/2(Lumda), 计算Cmz/2(Lumda), 计算Cmy/2(Lumda), 计算Cmx/2(Lumda), 计算Ctz/2(Lumda)  "<Lumda>"
  计算Ctx/1(Ctx) -> Mux/1  "Ctx"
  计算Cty/1(Cty) -> Mux/2  "Cty"
  计算Ctz/1(Ctz) -> Mux/3  "Ctz"
  计算Cmx/1(Cmx) -> Mux/4  "Cmx"
  计算Cmy/1(Cmy) -> Mux/5  "Cmy"
  计算Cmz/1(Cmz) -> Mux/6  "Cmz"
  Mux/1 -> Out1/1

== system test_bu01_2018b_tuning/Plant/bu01_model/动力系统模型/Motor2_TM_N/TM1654N /螺旋桨模型/螺旋桨气动/计算螺旋桨气动系数 ==
  In1 : Inport
  Bus Selector : BusSelector  OutputSignals=Miu,Lumda
  Mux : Mux  Inputs=6
  计算Cmx : Subsystem
  计算Cmy : Subsystem
  计算Cmz : Subsystem
  计算Ctx : Subsystem
  计算Cty : Subsystem
  计算Ctz : Subsystem
  Out1 : Outport
  wires:
  In1/1 -> Bus Selector/1
  Bus Selector/1 -> 计算Cmz/1(Miu), 计算Cmy/1(Miu), 计算Cmx/1(Miu), 计算Ctz/1(Miu), 计算Cty/1(Miu), 计算Ctx/1(Miu)  "<Miu>"
  Bus Selector/2 -> 计算Cmz/2(Lumda), 计算Cmy/2(Lumda), 计算Cmx/2(Lumda), 计算Ctz/2(Lumda), 计算Ctx/2(Lumda), 计算Cty/2(Lumda)  "<Lumda>"
  计算Ctx/1(Ctx) -> Mux/1  "Ctx"
  计算Cty/1(Cty) -> Mux/2  "Cty"
  计算Ctz/1(Ctz) -> Mux/3  "Ctz"
  计算Cmx/1(Cmx) -> Mux/4  "Cmx"
  计算Cmy/1(Cmy) -> Mux/5  "Cmy"
  计算Cmz/1(Cmz) -> Mux/6  "Cmz"
  Mux/1 -> Out1/1

== system test_bu01_2018b_tuning/Plant/bu01_model/动力系统模型/Motor3_TM_P/TM1654P /螺旋桨模型/螺旋桨气动/计算螺旋桨气动系数 ==
  In1 : Inport
  Bus Selector : BusSelector  OutputSignals=Miu,Lumda
  Mux : Mux  Inputs=6
  计算Cmx : Subsystem
  计算Cmy : Subsystem
  计算Cmz : Subsystem
  计算Ctx : Subsystem  TreatAsAtomicUnit=on
  计算Cty : Subsystem
  计算Ctz : Subsystem
  Out1 : Outport
  wires:
  In1/1 -> Bus Selector/1
  Bus Selector/1 -> 计算Ctz/1(Miu), 计算Cmz/1(Miu), 计算Cmy/1(Miu), 计算Cmx/1(Miu), 计算Cty/1(Miu), 计算Ctx/1(Miu)  "<Miu>"
  Bus Selector/2 -> 计算Cty/2(Lumda), 计算Ctx/2(Lumda), 计算Cmz/2(Lumda), 计算Cmy/2(Lumda), 计算Cmx/2(Lumda), 计算Ctz/2(Lumda)  "<Lumda>"
  计算Ctx/1(Ctx) -> Mux/1  "Ctx"
  计算Cty/1(Cty) -> Mux/2  "Cty"
  计算Ctz/1(Ctz) -> Mux/3  "Ctz"
  计算Cmx/1(Cmx) -> Mux/4  "Cmx"
  计算Cmy/1(Cmy) -> Mux/5  "Cmy"
  计算Cmz/1(Cmz) -> Mux/6  "Cmz"
  Mux/1 -> Out1/1
